simulink model "example_CondensingBoilerCONF"  (R2016b)
settings: Solver=ode45  StartTime=0.0  StopTime=1*24*3600  MaxStep=1800  RelTol=1e-4  AbsTol=1e-5  EnableMultiTasking=on
undefined symbols (not defined in the file): path_carnot
libraries: carnot x6, simulink x1
settings Model: Creator=drhf  LastModifiedBy=drhf
settings DataIOCC: LimitDataPoints=on  SaveFormat=Array  SignalLoggingSaveFormat=ModelDataLogs
settings OptimizationCC: ExpressionDepthLimit=2147483647  LifeSpan=inf
settings DebuggingCC: UnderspecifiedInitializationDetection=Classic  MergeDetectMultiDrivingBlocksExec=none  SolverPrmCheckMsg=warning  FcnCallInpInsideContextMsg=warning  StateNameClashWarn=warning  SFUnexpectedBacktrackingDiag=warning  SFNoUnconditionalDefaultTransitionDiag=warning  SFExecutionAtInitializationDiag=none
settings HardwareCC: ProdBitPerPointer=32  ProdBitPerSizeT=32  ProdBitPerPtrDiffT=32  ProdLargestAtomicFloat=None  ProdIntDivRoundTo=Undefined  ProdEndianess=Unspecified  ProdWordSize=32  ProdHWDeviceType=32-bit Generic
settings ModelReferenceCC: PropagateSignalLabelsOutOfModel=off
settings GRTTargetCC: TargetLangStandard=C89/C90 (ANSI)  GeneratePreprocessorConditionals=Disable all  CombineOutputUpdateFcns=off  GRTInterface=on
settings ConfigComp: CovMetricSettings=dw  CovHtmlReporting=on  CovSaveCumulativeToWorkspaceVar=on  CovSaveSingleToWorkspaceVar=on  CovExternalEMLEnable=off

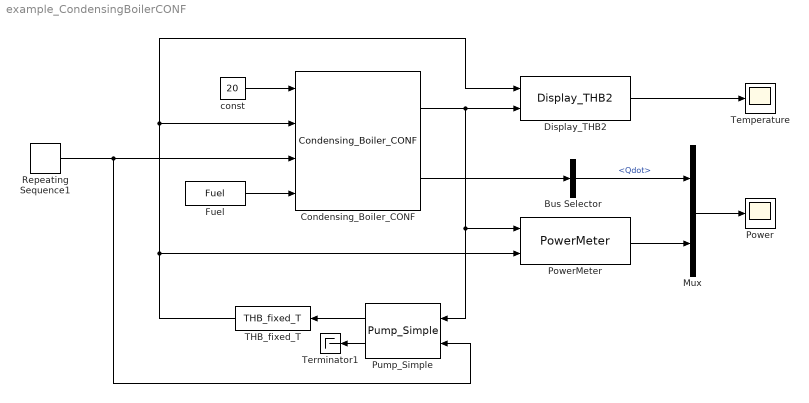
== system example_CondensingBoilerCONF ==
  Bus Selector : BusSelector  OutputSignals=Qdot
  Condensing_Boiler_CONF : carnot/Source/Boiler/Condensing_Boiler_CONF  Tini=20  PathName=fullfile(path_carnot('libsl'), 'Source','Boiler','Condensing_Boiler_CONF','parameter_set')  FileName='DefaultCondensingBoiler.mat'  userPath=off  userParam=off  Pgas=20000  HeatLoss=2.5  Volume=0.0035  ElectricPower=[50 200]  TableRelativePower=[0.1 1]  whichTforEfficiency=mean of inlet and outlet temperature  TableData=[1 1;1 1]  TableTemperatures=[10 90]  relQdotMin=0.1  dplin=10  dpqua=100  Nodes=3
  Display_THB2 : carnot/Outputs/Display_THB2  t=on  m=off  p=off  id=off  mix=off  d=off
  Fuel : carnot/Source/Energy/Fuel  ft=1  t=20  ls=1  p=1e5  h_values=[5.14e7 5.69e7]  tc=45  price=1  mass=[0.33 0.67 0 0 0 0]
  Mux : Mux  Inputs=2
  Power : Scope
  PowerMeter : carnot/Control/PowerMeter
  Pump_Simple : carnot/Hydraulics/Pump_Simple  mdotmax=2000/3600  dia=0.0157  power=30  fluid_id=Water  mix=0  p0=3e5
  Repeating Sequence1 : simulink/Sources/Repeating Sequence  rep_seq_t=[0 6 12]*3600  rep_seq_y=[0.1 1 0.1]
  THB_fixed_T : carnot/Source/Simple/THB_fixed_T  t=40
  Temperature : Scope
  Terminator1 : Terminator
  const : Constant  Value=20
  wires:
  const/1 -> Condensing_Boiler_CONF/1
  THB_fixed_T/1 -> PowerMeter/2, Condensing_Boiler_CONF/2, Display_THB2/1
  Repeating Sequence1/1 -> Condensing_Boiler_CONF/3, Pump_Simple/2
  Fuel/1 -> Condensing_Boiler_CONF/4
  Condensing_Boiler_CONF/1 -> PowerMeter/1, Pump_Simple/1, Display_THB2/2
  Display_THB2/1 -> Temperature/1
  Condensing_Boiler_CONF/2 -> Bus Selector/1
  Mux/1 -> Power/1
  PowerMeter/1 -> Mux/2
  Bus Selector/1 -> Mux/1  "<Qdot>"
  Pump_Simple/1 -> THB_fixed_T/1
  Pump_Simple/2 -> Terminator1/1
